simulink model "Logic_Final_Project_PRODUCT4_QUESTION37"  (R2025b)
settings: Solver=VariableStepAuto  StartTime=0.0  StopTime=100  RelTol=1e-3
libraries: simulink_extras x83
(part 1 of 2)
settings Model: Creator=60nur  LastModifiedBy=yusuf

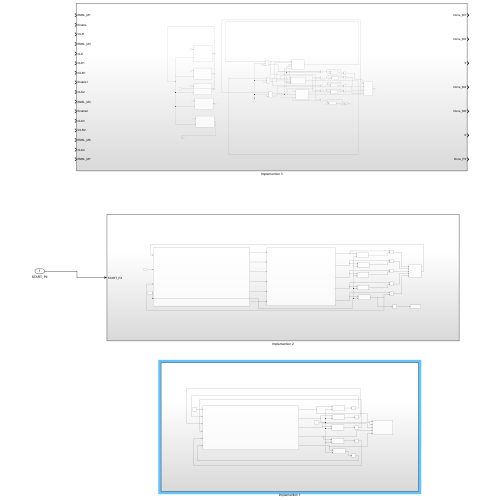
[thumbnail: Simulink's stored preview of the top-level diagram]
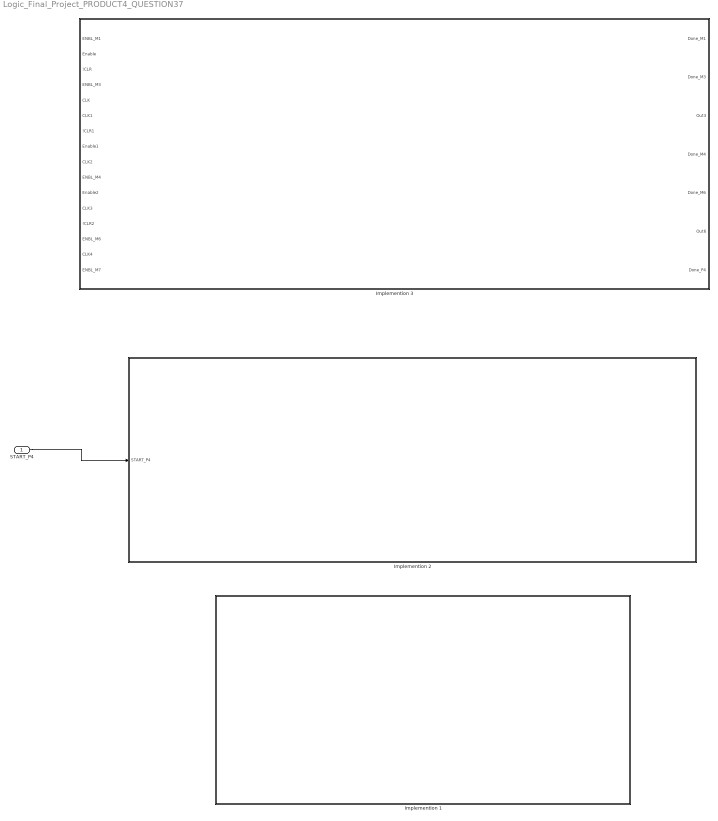
== system Logic_Final_Project_PRODUCT4_QUESTION37 ==
  START_P4 : Inport
  Implemention 1 : Subsystem
  Implemention 2 : Subsystem
  Implemention 3 : Subsystem
  wires:
  START_P4/1 -> Implemention 2/1(START_P4)

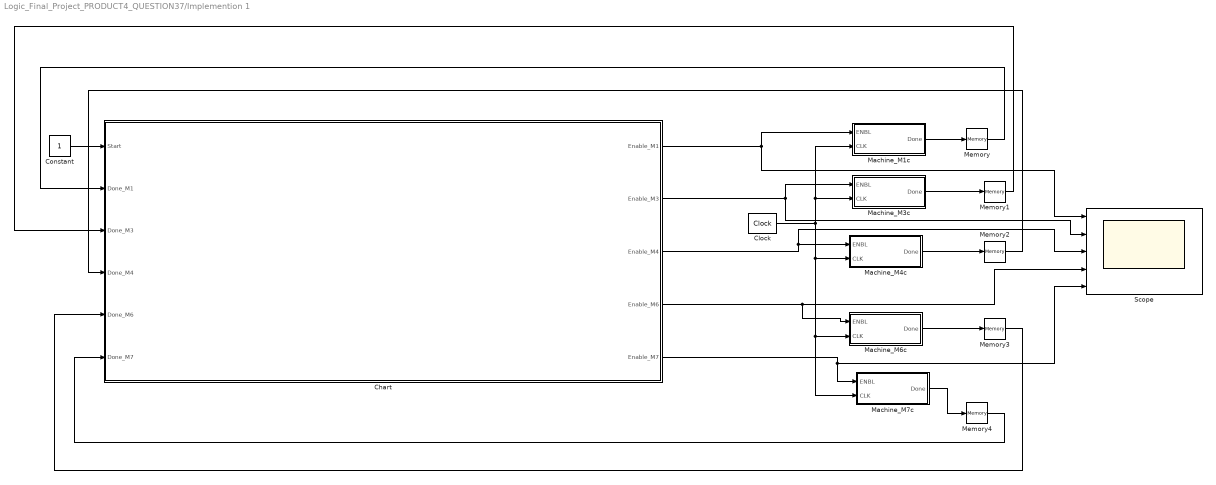
== system Logic_Final_Project_PRODUCT4_QUESTION37/Implemention 1 ==
  Chart : Stateflow chart  TreatAsAtomicUnit=on
  Clock : simulink_extras/Flip Flops/Clock  period=1
  Constant : Constant
  Machine_M1c : Subsystem
  Machine_M3c : Subsystem
  Machine_M4c : Subsystem
  Machine_M6c : Subsystem
  Machine_M7c : Subsystem
  Memory{,1..4} (5 alike) : Memory
  Scope : Scope  NumInputPorts=5
      settings: ActiveDisplayYMinimum=-0.1598262181001921  ActiveDisplayYMaximum=0.46246359997809955
  wires:
  Chart/5(Enable_M7) -> Machine_M7c/1(ENBL), Scope/5
  Chart/3(Enable_M4) -> Machine_M4c/1(ENBL), Scope/3
  Chart/4(Enable_M6) -> Machine_M6c/1(ENBL), Scope/4
  Memory3/1 -> Chart/5(Done_M6)
  Machine_M4c/1(Done) -> Memory2/1
  Machine_M3c/1(Done) -> Memory1/1
  Memory1/1 -> Chart/3(Done_M3)
  Memory4/1 -> Chart/6(Done_M7)
  Chart/2(Enable_M3) -> Machine_M3c/1(ENBL), Scope/2
  Chart/1(Enable_M1) -> Machine_M1c/1(ENBL), Scope/1
  Machine_M1c/1(Done) -> Memory/1
  Memory2/1 -> Chart/4(Done_M4)
  Clock/1 -> Machine_M1c/2(CLK), Machine_M3c/2(CLK), Machine_M7c/2(CLK), Machine_M6c/2(CLK), Machine_M4c/2(CLK)
  Constant/1 -> Chart/1(Start)
  Memory/1 -> Chart/2(Done_M1)
  Machine_M7c/1(Done) -> Memory4/1
  Machine_M6c/1(Done) -> Memory3/1

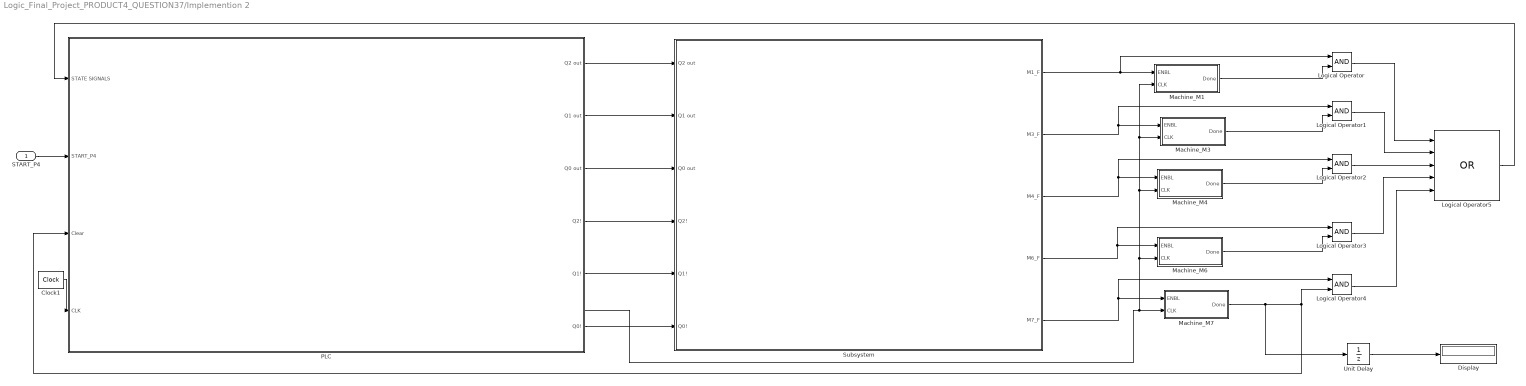
== system Logic_Final_Project_PRODUCT4_QUESTION37/Implemention 2 ==
  START_P4 : Inport
  Clock1 : simulink_extras/Flip Flops/Clock  period=1
  Display : Display
  Logical Operator{,1..4} (5 alike) : Logic  AllPortsSameDT=off  OutDataTypeStr=boolean
  Logical Operator5 : Logic  Operator=OR  Inputs=5  AllPortsSameDT=off  OutDataTypeStr=boolean
  Machine_M1 : Subsystem
  Machine_M3 : Subsystem
  Machine_M4 : Subsystem
  Machine_M6 : Subsystem
  Machine_M7 : Subsystem
  PLC : Subsystem
  Subsystem : Subsystem
  Unit Delay : UnitDelay  SampleTime=-1  HasFrameUpgradeWarning=on
  wires:
  Clock1/1 -> PLC/4(CLK), Machine_M6/2(CLK), Machine_M1/2(CLK), Machine_M3/2(CLK), Machine_M4/2(CLK), Machine_M7/2(CLK)
  PLC/1(Q2 out) -> Subsystem/1(Q2 out)
  Machine_M6/1(Done) -> Logical Operator3/2
  Subsystem/1(M1_F) -> Logical Operator/1, Machine_M1/1(ENBL)
  Subsystem/2(M3_F) -> Logical Operator1/1, Machine_M3/1(ENBL)
  Logical Operator/1 -> Logical Operator5/1
  Machine_M7/1(Done) -> Unit Delay/1, PLC/3(Clear), Logical Operator4/2
  Logical Operator4/1 -> Logical Operator5/5
  Logical Operator2/1 -> Logical Operator5/3
  Logical Operator3/1 -> Logical Operator5/4
  PLC/2(Q1 out) -> Subsystem/2(Q1 out)
  PLC/6(Q0!) -> Subsystem/6(Q0!)
  Unit Delay/1 -> Display/1
  Machine_M4/1(Done) -> Logical Operator2/2
  Subsystem/5(M7_F) -> Logical Operator4/1, Machine_M7/1(ENBL)
  PLC/5(Q1!) -> Subsystem/5(Q1!)
  Subsystem/3(M4_F) -> Logical Operator2/1, Machine_M4/1(ENBL)
  Subsystem/4(M6_F) -> Logical Operator3/1, Machine_M6/1(ENBL)
  PLC/4(Q2!) -> Subsystem/4(Q2!)
  PLC/3(Q0 out) -> Subsystem/3(Q0 out)
  START_P4/1 -> PLC/2(START_P4)
  Machine_M3/1(Done) -> Logical Operator1/2
  Logical Operator1/1 -> Logical Operator5/2
  Machine_M1/1(Done) -> Logical Operator/2
  Logical Operator5/1 -> PLC/1("STATE SIGNALS ")

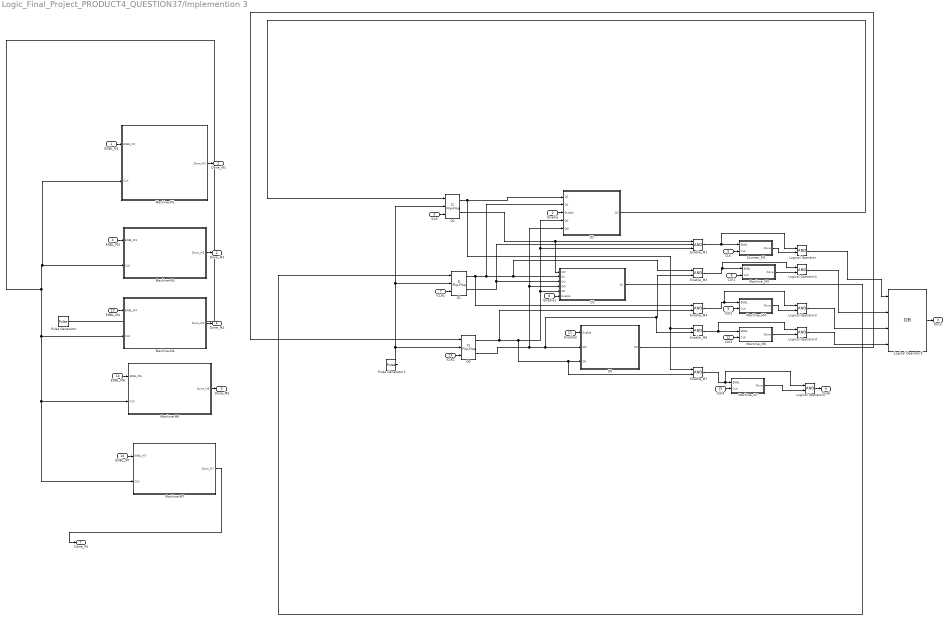
== system Logic_Final_Project_PRODUCT4_QUESTION37/Implemention 3 ==
  ENBL_M1 : Inport
  Enable : Inport  Port=2
  !CLR : Inport  Port=3
  ENBL_M3 : Inport  Port=4
  CLK : Inport  Port=5
  CLK1 : Inport  Port=6
  !CLR1 : Inport  Port=7
  Enable1 : Inport  Port=8
  CLK2 : Inport  Port=9
  ENBL_M4 : Inport  Port=10
  Enable2 : Inport  Port=11
  CLK3 : Inport  Port=12
  !CLR2 : Inport  Port=13
  ENBL_M6 : Inport  Port=14
  CLK4 : Inport  Port=15
  ENBL_M7 : Inport  Port=16
  Counter_M1 : Subsystem
  D0 : Subsystem
  D1 : Subsystem
  "D2 " : Subsystem
  Enable_M1 : Logic  Inputs=3  AllPortsSameDT=off  OutDataTypeStr=boolean
  Enable_M{3..4,6..7} (4 alike) : Logic  AllPortsSameDT=off  OutDataTypeStr=boolean
  Logical Operator{,1..4} (5 alike) : Logic  AllPortsSameDT=off  OutDataTypeStr=boolean
  Logical Operator5 : Logic  Operator=OR  Inputs=4  AllPortsSameDT=off  OutDataTypeStr=boolean
  Machine-M1 : Subsystem
  Machine-M3 : Subsystem
  Machine-M4 : Subsystem
  Machine-M6 : Subsystem
  Machine-M7 : Subsystem
  Machine_M3 : Subsystem
  Machine_M4 : Subsystem
  Machine_M6 : Subsystem
  Machine_M7 : Subsystem
  Pulse Generator : DiscretePulseGenerator  Period=10  PulseWidth=5  SampleTime=-1
  Pulse Generator1 : DiscretePulseGenerator  Period=10  PulseWidth=5  SampleTime=-1
  Q0 : simulink_extras/Flip Flops/D Flip-Flop
  Q1 : simulink_extras/Flip Flops/D Flip-Flop
  Q2 : simulink_extras/Flip Flops/D Flip-Flop
  Done_M1 : Outport
  Done_M3 : Outport  Port=2
  Out3 : Outport  Port=3
  Done_M4 : Outport  Port=4
  Done_M6 : Outport  Port=5
  Out6 : Outport  Port=6
  Done_P4 : Outport  Port=7
  wires:
  Machine_M7/1(Done) -> Logical Operator4/2
  Pulse Generator/1 -> Machine-M1/2(CLK), Machine-M3/2(CLK), Machine-M4/2(CLK), Machine-M7/2(CLK), Machine-M6/2(CLK)
  Q0/1 -> Enable_M4/2, D1/5(Q0), Enable_M1/3, "D2 "/4(Q0), Enable_M7/2, D0/3(Q0)
  Q2/1 -> Enable_M6/1, Enable_M7/1, "D2 "/1(Q2)
  Q1/1 -> Enable_M4/1, Enable_M3/1, D1/2(Q1), "D2 "/2(Q1)
  Enable_M7/1 -> Logical Operator4/1, Machine_M7/1(ENBL)
  Logical Operator2/1 -> Logical Operator5/3
  Machine_M6/1(Done) -> Logical Operator3/2
  Q1/2 -> Enable_M1/2, D1/3(Q1!)
  CLK4/1 -> Machine_M7/2(CLK)
  Enable_M3/1 -> Logical Operator1/1, Machine_M3/1(ENBL)
  Q2/2 -> Enable_M1/1, D1/1(Q2!)
  Logical Operator/1 -> Logical Operator5/1
  Machine-M7/1(Done_M7) -> Done_P4/1
  Enable_M4/1 -> Logical Operator2/1, Machine_M4/1(ENBL)
  Machine_M3/1(Done) -> Logical Operator1/2
  Pulse Generator1/1 -> Q0/2, Q1/2, Q2/2
  Enable/1 -> "D2 "/3(Enable)
  "D2 "/1(D2) -> Q2/1
  Machine-M3/1(Done_M3) -> Done_M3/1
  ENBL_M3/1 -> Machine-M3/1(ENBL_M3)
  D1/1(D1) -> Q1/1
  D0/1(D0) -> Q0/1
  Enable_M6/1 -> Logical Operator3/1, Machine_M6/1(ENBL)
  ENBL_M4/1 -> Machine-M4/1(ENBL_M4)
  Logical Operator5/1 -> Out3/1
  Counter_M1/1(Done) -> Logical Operator/2
  Enable_M1/1 -> Logical Operator/1, Counter_M1/1(ENBL)
  Logical Operator1/1 -> Logical Operator5/2
  ENBL_M1/1 -> Machine-M1/1(ENBL_M1)
  Machine_M4/1(Done) -> Logical Operator2/2
  Logical Operator3/1 -> Logical Operator5/4
  Q0/2 -> D0/2(Q0!), Enable_M6/2, Enable_M3/2, "D2 "/5(Q0!), D1/4(Q0!)
  CLK/1 -> Counter_M1/2(CLK)
  ENBL_M6/1 -> Machine-M6/1(ENBL_M6)
  CLK1/1 -> Machine_M3/2(CLK)
  Enable2/1 -> D0/1(Enable)
  !CLR1/1 -> Q1/3
  Machine-M6/1(Done_M6) -> Done_M6/1
  !CLR/1 -> Q2/3
  !CLR2/1 -> Q0/3
  Machine-M1/1(Done_M1) -> Done_M1/1
  Enable1/1 -> D1/6(Enable)
  CLK2/1 -> Machine_M4/2(CLK)
  Machine-M4/1(Done_M4) -> Done_M4/1
  CLK3/1 -> Machine_M6/2(CLK)
  ENBL_M7/1 -> Machine-M7/1(ENBL_M7)
  Logical Operator4/1 -> Out6/1

== system Logic_Final_Project_PRODUCT4_QUESTION37/Implemention 1/Machine_M1c ==
  ENBL : Inport
  CLK : Inport  Port=2
  D Flip-Flop 0 : simulink_extras/Flip Flops/D Flip-Flop
  D Flip-Flop1 : simulink_extras/Flip Flops/D Flip-Flop
  D Flip-Flop2 : simulink_extras/Flip Flops/D Flip-Flop
  Logical Operator : Logic  Operator=XOR  AllPortsSameDT=off  OutDataTypeStr=boolean
  Logical Operator1 : Logic  AllPortsSameDT=off  OutDataTypeStr=boolean
  Logical Operator2 : Logic  AllPortsSameDT=off  OutDataTypeStr=boolean
  Logical Operator3 : Logic  Operator=XOR  AllPortsSameDT=off  OutDataTypeStr=boolean
  Done : Outport
  wires:
  D Flip-Flop 0/2 -> D Flip-Flop 0/1
  D Flip-Flop 0/1 -> Logical Operator1/1, Logical Operator/1, Logical Operator2/1
  D Flip-Flop1/1 -> Logical Operator1/2, Logical Operator/2
  Logical Operator/1 -> D Flip-Flop1/1
  Logical Operator1/1 -> Logical Operator3/1
  D Flip-Flop2/1 -> Logical Operator2/2, Logical Operator3/2
  Logical Operator3/1 -> D Flip-Flop2/1
  ENBL/1 -> D Flip-Flop 0/3, D Flip-Flop2/3, D Flip-Flop1/3
  CLK/1 -> D Flip-Flop 0/2, D Flip-Flop1/2, D Flip-Flop2/2
  Logical Operator2/1 -> Done/1

== system Logic_Final_Project_PRODUCT4_QUESTION37/Implemention 1/Machine_M3c ==
  ENBL : Inport
  CLK : Inport  Port=2
  D Flip-Flop 0 : simulink_extras/Flip Flops/D Flip-Flop
  D Flip-Flop1 : simulink_extras/Flip Flops/D Flip-Flop
  D Flip-Flop2 : simulink_extras/Flip Flops/D Flip-Flop
  Logical Operator : Logic  Operator=XOR  AllPortsSameDT=off  OutDataTypeStr=boolean
  Logical Operator1 : Logic  AllPortsSameDT=off  OutDataTypeStr=boolean
  Logical Operator3 : Logic  Operator=XOR  AllPortsSameDT=off  OutDataTypeStr=boolean
  Done : Outport
  wires:
  CLK/1 -> D Flip-Flop2/2, D Flip-Flop1/2, D Flip-Flop 0/2
  ENBL/1 -> D Flip-Flop1/3, D Flip-Flop2/3, D Flip-Flop 0/3
  Logical Operator3/1 -> D Flip-Flop2/1
  D Flip-Flop2/1 -> Done/1, Logical Operator3/2
  Logical Operator1/1 -> Logical Operator3/1
  Logical Operator/1 -> D Flip-Flop1/1
  D Flip-Flop1/1 -> Logical Operator/2, Logical Operator1/2
  D Flip-Flop 0/1 -> Logical Operator/1, Logical Operator1/1
  D Flip-Flop 0/2 -> D Flip-Flop 0/1

== system Logic_Final_Project_PRODUCT4_QUESTION37/Implemention 1/Machine_M4c ==
  ENBL : Inport
  CLK : Inport  Port=2
  D Flip-Flop 0 : simulink_extras/Flip Flops/D Flip-Flop
  D Flip-Flop1 : simulink_extras/Flip Flops/D Flip-Flop
  D Flip-Flop2 : simulink_extras/Flip Flops/D Flip-Flop
  Logical Operator : Logic  Operator=XOR  AllPortsSameDT=off  OutDataTypeStr=boolean
  Logical Operator1 : Logic  AllPortsSameDT=off  OutDataTypeStr=boolean
  Logical Operator2 : Logic  AllPortsSameDT=off  OutDataTypeStr=boolean
  Logical Operator3 : Logic  Operator=XOR  AllPortsSameDT=off  OutDataTypeStr=boolean
  Done : Outport
  wires:
  Logical Operator2/1 -> Done/1
  CLK/1 -> D Flip-Flop2/2, D Flip-Flop1/2, D Flip-Flop 0/2
  ENBL/1 -> D Flip-Flop1/3, D Flip-Flop2/3, D Flip-Flop 0/3
  Logical Operator3/1 -> D Flip-Flop2/1
  D Flip-Flop2/1 -> Logical Operator3/2, Logical Operator2/2
  Logical Operator1/1 -> Logical Operator3/1
  Logical Operator/1 -> D Flip-Flop1/1
  D Flip-Flop1/1 -> Logical Operator/2, Logical Operator1/2
  D Flip-Flop 0/1 -> Logical Operator2/1, Logical Operator/1, Logical Operator1/1
  D Flip-Flop 0/2 -> D Flip-Flop 0/1

== system Logic_Final_Project_PRODUCT4_QUESTION37/Implemention 1/Machine_M6c ==
  ENBL : Inport
  CLK : Inport  Port=2
  D Flip-Flop 0 : simulink_extras/Flip Flops/D Flip-Flop
  D Flip-Flop1 : simulink_extras/Flip Flops/D Flip-Flop
  D Flip-Flop2 : simulink_extras/Flip Flops/D Flip-Flop
  Logical Operator : Logic  Operator=XOR  AllPortsSameDT=off  OutDataTypeStr=boolean
  Logical Operator1 : Logic  AllPortsSameDT=off  OutDataTypeStr=boolean
  Logical Operator2 : Logic  AllPortsSameDT=off  OutDataTypeStr=boolean
  Logical Operator3 : Logic  Operator=XOR  AllPortsSameDT=off  OutDataTypeStr=boolean
  Done : Outport
  wires:
  Logical Operator2/1 -> Done/1
  CLK/1 -> D Flip-Flop2/2, D Flip-Flop1/2, D Flip-Flop 0/2
  ENBL/1 -> D Flip-Flop1/3, D Flip-Flop2/3, D Flip-Flop 0/3
  Logical Operator3/1 -> D Flip-Flop2/1
  D Flip-Flop2/1 -> Logical Operator3/2, Logical Operator2/2
  Logical Operator1/1 -> Logical Operator3/1
  Logical Operator/1 -> D Flip-Flop1/1
  D Flip-Flop1/1 -> Logical Operator/2, Logical Operator1/2, Logical Operator2/1
  D Flip-Flop 0/1 -> Logical Operator/1, Logical Operator1/1
  D Flip-Flop 0/2 -> D Flip-Flop 0/1

== system Logic_Final_Project_PRODUCT4_QUESTION37/Implemention 1/Machine_M7c ==
  ENBL : Inport
  CLK : Inport  Port=2
  D Flip-Flop 0 : simulink_extras/Flip Flops/D Flip-Flop
  D Flip-Flop1 : simulink_extras/Flip Flops/D Flip-Flop
  D Flip-Flop2 : simulink_extras/Flip Flops/D Flip-Flop
  Logical Operator : Logic  Operator=XOR  AllPortsSameDT=off  OutDataTypeStr=boolean
  Logical Operator1 : Logic  AllPortsSameDT=off  OutDataTypeStr=boolean
  Logical Operator3 : Logic  Operator=XOR  AllPortsSameDT=off  OutDataTypeStr=boolean
  Done : Outport
  wires:
  D Flip-Flop 0/2 -> D Flip-Flop 0/1
  D Flip-Flop 0/1 -> Logical Operator1/1, Logical Operator/1
  D Flip-Flop1/1 -> Done/1, Logical Operator1/2, Logical Operator/2
  Logical Operator/1 -> D Flip-Flop1/1
  Logical Operator1/1 -> Logical Operator3/1
  D Flip-Flop2/1 -> Logical Operator3/2
  Logical Operator3/1 -> D Flip-Flop2/1
  ENBL/1 -> D Flip-Flop 0/3, D Flip-Flop2/3, D Flip-Flop1/3
  CLK/1 -> D Flip-Flop 0/2, D Flip-Flop1/2, D Flip-Flop2/2

== system Logic_Final_Project_PRODUCT4_QUESTION37/Implemention 2/Machine_M1 ==
  ENBL : Inport
  CLK : Inport  Port=2
  D Flip-Flop 0 : simulink_extras/Flip Flops/D Flip-Flop
  D Flip-Flop1 : simulink_extras/Flip Flops/D Flip-Flop
  D Flip-Flop2 : simulink_extras/Flip Flops/D Flip-Flop
  Logical Operator : Logic  Operator=XOR  AllPortsSameDT=off  OutDataTypeStr=boolean
  Logical Operator1 : Logic  AllPortsSameDT=off  OutDataTypeStr=boolean
  Logical Operator2 : Logic  AllPortsSameDT=off  OutDataTypeStr=boolean
  Logical Operator3 : Logic  Operator=XOR  AllPortsSameDT=off  OutDataTypeStr=boolean
  Done : Outport
  wires:
  D Flip-Flop 0/2 -> D Flip-Flop 0/1
  D Flip-Flop 0/1 -> Logical Operator1/1, Logical Operator/1, Logical Operator2/1
  D Flip-Flop1/1 -> Logical Operator1/2, Logical Operator/2
  Logical Operator/1 -> D Flip-Flop1/1
  Logical Operator1/1 -> Logical Operator3/1
  D Flip-Flop2/1 -> Logical Operator2/2, Logical Operator3/2
  Logical Operator3/1 -> D Flip-Flop2/1
  ENBL/1 -> D Flip-Flop 0/3, D Flip-Flop2/3, D Flip-Flop1/3
  CLK/1 -> D Flip-Flop 0/2, D Flip-Flop1/2, D Flip-Flop2/2
  Logical Operator2/1 -> Done/1

== system Logic_Final_Project_PRODUCT4_QUESTION37/Implemention 2/Machine_M3 ==
  ENBL : Inport
  CLK : Inport  Port=2
  D Flip-Flop 0 : simulink_extras/Flip Flops/D Flip-Flop
  D Flip-Flop1 : simulink_extras/Flip Flops/D Flip-Flop
  D Flip-Flop2 : simulink_extras/Flip Flops/D Flip-Flop
  Logical Operator : Logic  Operator=XOR  AllPortsSameDT=off  OutDataTypeStr=boolean
  Logical Operator1 : Logic  AllPortsSameDT=off  OutDataTypeStr=boolean
  Logical Operator3 : Logic  Operator=XOR  AllPortsSameDT=off  OutDataTypeStr=boolean
  Done : Outport
  wires:
  CLK/1 -> D Flip-Flop2/2, D Flip-Flop1/2, D Flip-Flop 0/2
  ENBL/1 -> D Flip-Flop1/3, D Flip-Flop2/3, D Flip-Flop 0/3
  Logical Operator3/1 -> D Flip-Flop2/1
  D Flip-Flop2/1 -> Done/1, Logical Operator3/2
  Logical Operator1/1 -> Logical Operator3/1
  Logical Operator/1 -> D Flip-Flop1/1
  D Flip-Flop1/1 -> Logical Operator/2, Logical Operator1/2
  D Flip-Flop 0/1 -> Logical Operator/1, Logical Operator1/1
  D Flip-Flop 0/2 -> D Flip-Flop 0/1

== system Logic_Final_Project_PRODUCT4_QUESTION37/Implemention 2/Machine_M4 ==
  ENBL : Inport
  CLK : Inport  Port=2
  D Flip-Flop 0 : simulink_extras/Flip Flops/D Flip-Flop
  D Flip-Flop1 : simulink_extras/Flip Flops/D Flip-Flop
  D Flip-Flop2 : simulink_extras/Flip Flops/D Flip-Flop
  Logical Operator : Logic  Operator=XOR  AllPortsSameDT=off  OutDataTypeStr=boolean
  Logical Operator1 : Logic  AllPortsSameDT=off  OutDataTypeStr=boolean
  Logical Operator2 : Logic  AllPortsSameDT=off  OutDataTypeStr=boolean
  Logical Operator3 : Logic  Operator=XOR  AllPortsSameDT=off  OutDataTypeStr=boolean
  Done : Outport
  wires:
  Logical Operator2/1 -> Done/1
  CLK/1 -> D Flip-Flop2/2, D Flip-Flop1/2, D Flip-Flop 0/2
  ENBL/1 -> D Flip-Flop1/3, D Flip-Flop2/3, D Flip-Flop 0/3
  Logical Operator3/1 -> D Flip-Flop2/1
  D Flip-Flop2/1 -> Logical Operator3/2, Logical Operator2/2
  Logical Operator1/1 -> Logical Operator3/1
  Logical Operator/1 -> D Flip-Flop1/1
  D Flip-Flop1/1 -> Logical Operator/2, Logical Operator1/2
  D Flip-Flop 0/1 -> Logical Operator2/1, Logical Operator/1, Logical Operator1/1
  D Flip-Flop 0/2 -> D Flip-Flop 0/1

== system Logic_Final_Project_PRODUCT4_QUESTION37/Implemention 2/Machine_M6 ==
  ENBL : Inport
  CLK : Inport  Port=2
  D Flip-Flop 0 : simulink_extras/Flip Flops/D Flip-Flop
  D Flip-Flop1 : simulink_extras/Flip Flops/D Flip-Flop
  D Flip-Flop2 : simulink_extras/Flip Flops/D Flip-Flop
  Logical Operator : Logic  Operator=XOR  AllPortsSameDT=off  OutDataTypeStr=boolean
  Logical Operator1 : Logic  AllPortsSameDT=off  OutDataTypeStr=boolean
  Logical Operator2 : Logic  AllPortsSameDT=off  OutDataTypeStr=boolean
  Logical Operator3 : Logic  Operator=XOR  AllPortsSameDT=off  OutDataTypeStr=boolean
  Done : Outport
  wires:
  Logical Operator2/1 -> Done/1
  CLK/1 -> D Flip-Flop2/2, D Flip-Flop1/2, D Flip-Flop 0/2
  ENBL/1 -> D Flip-Flop1/3, D Flip-Flop2/3, D Flip-Flop 0/3
  Logical Operator3/1 -> D Flip-Flop2/1
  D Flip-Flop2/1 -> Logical Operator3/2, Logical Operator2/2
  Logical Operator1/1 -> Logical Operator3/1
  Logical Operator/1 -> D Flip-Flop1/1
  D Flip-Flop1/1 -> Logical Operator/2, Logical Operator1/2, Logical Operator2/1
  D Flip-Flop 0/1 -> Logical Operator/1, Logical Operator1/1
  D Flip-Flop 0/2 -> D Flip-Flop 0/1

== system Logic_Final_Project_PRODUCT4_QUESTION37/Implemention 2/Machine_M7 ==
  ENBL : Inport
  CLK : Inport  Port=2
  D Flip-Flop 0 : simulink_extras/Flip Flops/D Flip-Flop
  D Flip-Flop1 : simulink_extras/Flip Flops/D Flip-Flop
  D Flip-Flop2 : simulink_extras/Flip Flops/D Flip-Flop
  Logical Operator : Logic  Operator=XOR  AllPortsSameDT=off  OutDataTypeStr=boolean
  Logical Operator1 : Logic  AllPortsSameDT=off  OutDataTypeStr=boolean
  Logical Operator3 : Logic  Operator=XOR  AllPortsSameDT=off  OutDataTypeStr=boolean
  Unit Delay : UnitDelay  SampleTime=-1  HasFrameUpgradeWarning=on
  Done : Outport
  wires:
  D Flip-Flop 0/2 -> D Flip-Flop 0/1
  D Flip-Flop 0/1 -> Logical Operator1/1, Logical Operator/1
  Logical Operator1/1 -> Logical Operator3/1
  D Flip-Flop2/1 -> Logical Operator3/2
  Logical Operator3/1 -> D Flip-Flop2/1
  ENBL/1 -> D Flip-Flop 0/3, D Flip-Flop2/3, D Flip-Flop1/3
  CLK/1 -> D Flip-Flop 0/2, D Flip-Flop1/2, D Flip-Flop2/2
  Logical Operator/1 -> D Flip-Flop1/1
  D Flip-Flop1/1 -> Unit Delay/1
  Unit Delay/1 -> Done/1, Logical Operator/2, Logical Operator1/2

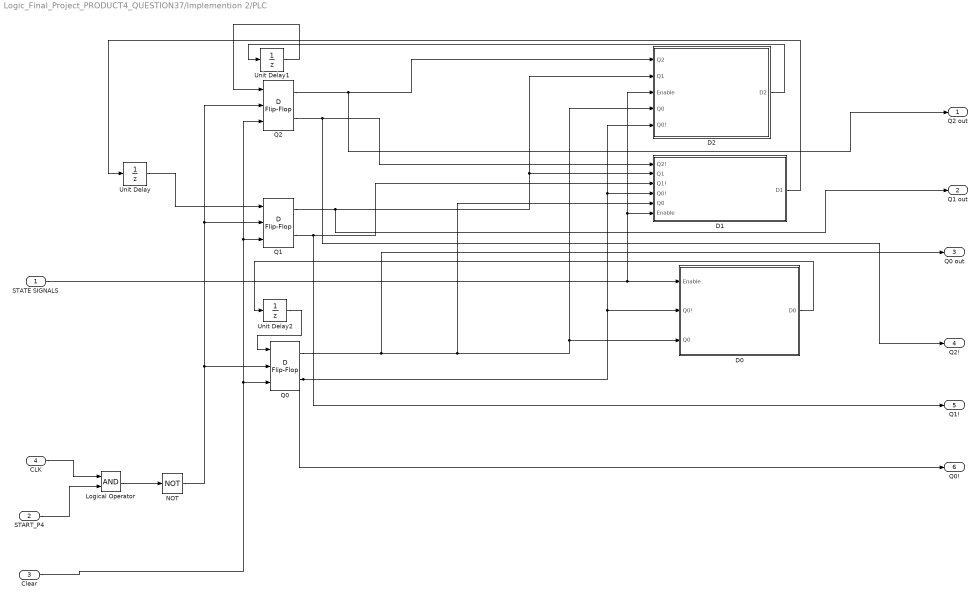
== system Logic_Final_Project_PRODUCT4_QUESTION37/Implemention 2/PLC ==
  "STATE SIGNALS " : Inport
  START_P4 : Inport  Port=2
  Clear : Inport  Port=3
  CLK : Inport  Port=4
  D0 : Subsystem
  D1 : Subsystem
  "D2 " : Subsystem
  Logical Operator : Logic  AllPortsSameDT=off  OutDataTypeStr=boolean
  NOT : Logic  Operator=NOT  IconShape=distinctive  AllPortsSameDT=off  OutDataTypeStr=boolean
  Q0 : simulink_extras/Flip Flops/D Flip-Flop
  Q1 : simulink_extras/Flip Flops/D Flip-Flop
  Q2 : simulink_extras/Flip Flops/D Flip-Flop
  Unit Delay : UnitDelay  SampleTime=-1  HasFrameUpgradeWarning=on
  Unit Delay1 : UnitDelay  SampleTime=-1  HasFrameUpgradeWarning=on
  Unit Delay2 : UnitDelay  SampleTime=-1  HasFrameUpgradeWarning=on
  Q2 out : Outport
  Q1 out : Outport  Port=2
  Q0 out : Outport  Port=3
  Q2! : Outport  Port=4
  Q1! : Outport  Port=5
  Q0! : Outport  Port=6
  wires:
  Q2/1 -> Q2 out/1, "D2 "/1(Q2)
  Q1/1 -> Q1 out/1, "D2 "/2(Q1), D1/2(Q1)
  Q0/1 -> Q0 out/1, D1/5(Q0), "D2 "/4(Q0), D0/3(Q0)
  Q0/2 -> Q0!/1, "D2 "/5(Q0!), D1/4(Q0!), D0/2(Q0!)
  Q2/2 -> Q2!/1, D1/1(Q2!)
  Q1/2 -> Q1!/1, D1/3(Q1!)
  Logical Operator/1 -> NOT/1
  CLK/1 -> Logical Operator/1
  NOT/1 -> Q0/2, Q2/2, Q1/2
  "STATE SIGNALS "/1 -> "D2 "/3(Enable), D1/6(Enable), D0/1(Enable)
  Clear/1 -> Q2/3, Q1/3, Q0/3
  Unit Delay2/1 -> Q0/1
  D0/1(D0) -> Unit Delay2/1
  Unit Delay1/1 -> Q2/1
  "D2 "/1(D2) -> Unit Delay1/1
  Unit Delay/1 -> Q1/1
  D1/1(D1) -> Unit Delay/1
  START_P4/1 -> Logical Operator/2

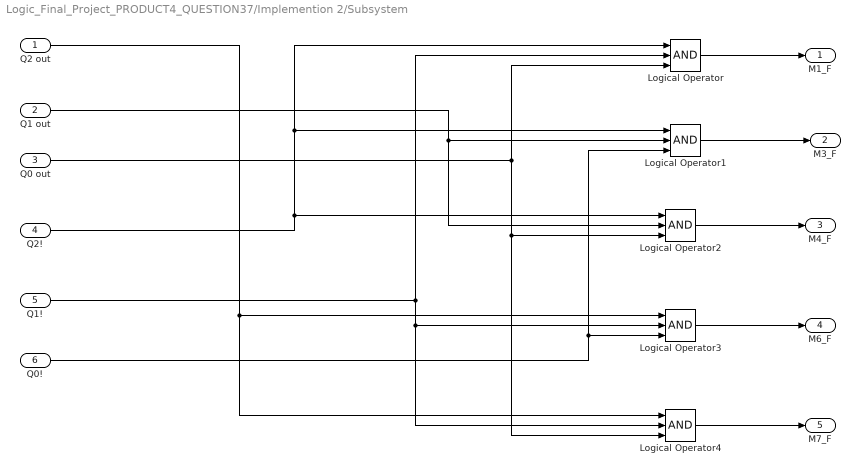
== system Logic_Final_Project_PRODUCT4_QUESTION37/Implemention 2/Subsystem ==
  Q2 out : Inport
  Q1 out : Inport  Port=2
  Q0 out : Inport  Port=3
  Q2! : Inport  Port=4
  Q1! : Inport  Port=5
  Q0! : Inport  Port=6
  Logical Operator{,1..4} (5 alike) : Logic  Inputs=3  AllPortsSameDT=off  OutDataTypeStr=boolean
  M1_F : Outport
  M3_F : Outport  Port=2
  M4_F : Outport  Port=3
  M6_F : Outport  Port=4
  M7_F : Outport  Port=5
  wires:
  Logical Operator2/1 -> M4_F/1
  Logical Operator4/1 -> M7_F/1
  Logical Operator3/1 -> M6_F/1
  Logical Operator1/1 -> M3_F/1
  Logical Operator/1 -> M1_F/1
  Q2!/1 -> Logical Operator2/1, Logical Operator1/1, Logical Operator/1
  Q1!/1 -> Logical Operator3/2, Logical Operator4/2, Logical Operator/2
  Q0 out/1 -> Logical Operator2/3, Logical Operator4/3, Logical Operator/3
  Q1 out/1 -> Logical Operator2/2, Logical Operator1/2
  Q0!/1 -> Logical Operator1/3, Logical Operator3/3
  Q2 out/1 -> Logical Operator4/1, Logical Operator3/1

== system Logic_Final_Project_PRODUCT4_QUESTION37/Implemention 3/Counter_M1 ==
  ENBL : Inport
  CLK : Inport  Port=2
  D Flip-Flop 0 : simulink_extras/Flip Flops/D Flip-Flop
  D Flip-Flop1 : simulink_extras/Flip Flops/D Flip-Flop
  D Flip-Flop2 : simulink_extras/Flip Flops/D Flip-Flop
  Logical Operator : Logic  Operator=XOR  AllPortsSameDT=off  OutDataTypeStr=boolean
  Logical Operator1 : Logic  AllPortsSameDT=off  OutDataTypeStr=boolean
  Logical Operator2 : Logic  AllPortsSameDT=off  OutDataTypeStr=boolean
  Logical Operator3 : Logic  Operator=XOR  AllPortsSameDT=off  OutDataTypeStr=boolean
  Done : Outport
  wires:
  D Flip-Flop 0/2 -> D Flip-Flop 0/1
  D Flip-Flop 0/1 -> Logical Operator1/1, Logical Operator/1, Logical Operator2/1
  D Flip-Flop1/1 -> Logical Operator1/2, Logical Operator/2
  Logical Operator/1 -> D Flip-Flop1/1
  Logical Operator1/1 -> Logical Operator3/1
  D Flip-Flop2/1 -> Logical Operator2/2, Logical Operator3/2
  Logical Operator3/1 -> D Flip-Flop2/1
  ENBL/1 -> D Flip-Flop 0/3, D Flip-Flop2/3, D Flip-Flop1/3
  CLK/1 -> D Flip-Flop 0/2, D Flip-Flop1/2, D Flip-Flop2/2
  Logical Operator2/1 -> Done/1

== system Logic_Final_Project_PRODUCT4_QUESTION37/Implemention 3/D0 ==
  Enable : Inport
  Q0! : Inport  Port=2
  Q0 : Inport  Port=3
  Logical Operator : Logic  AllPortsSameDT=off  OutDataTypeStr=boolean
  Logical Operator1 : Logic  Operator=NOT  AllPortsSameDT=off  OutDataTypeStr=boolean
  Logical Operator2 : Logic  Operator=OR  AllPortsSameDT=off  OutDataTypeStr=boolean
  Logical Operator3 : Logic  AllPortsSameDT=off  OutDataTypeStr=boolean
  D0 : Outport
  wires:
  Logical Operator1/1 -> Logical Operator/2
  Logical Operator/1 -> Logical Operator2/2
  Logical Operator2/1 -> D0/1
  Logical Operator3/1 -> Logical Operator2/1
  Enable/1 -> Logical Operator1/1, Logical Operator3/1
  Q0!/1 -> Logical Operator3/2
  Q0/1 -> Logical Operator/1

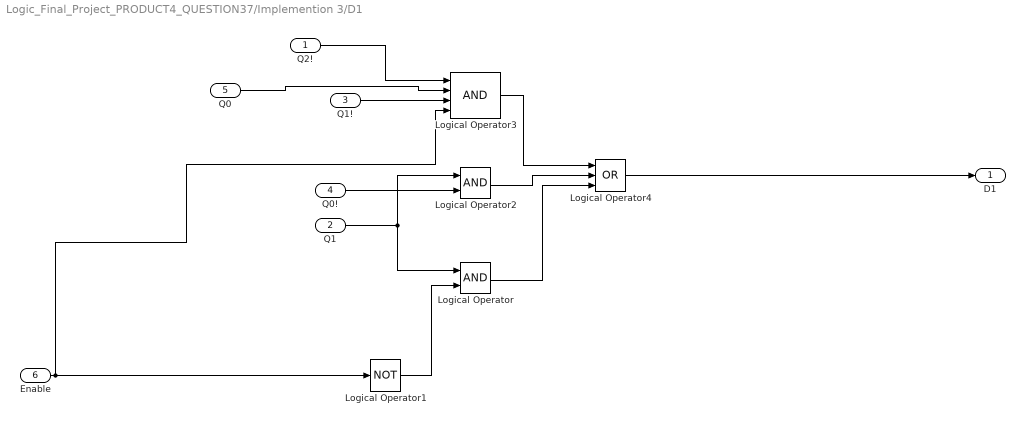
== system Logic_Final_Project_PRODUCT4_QUESTION37/Implemention 3/D1 ==
  Q2! : Inport
  Q1 : Inport  Port=2
  Q1! : Inport  Port=3
  Q0! : Inport  Port=4
  Q0 : Inport  Port=5
  Enable : Inport  Port=6
  Logical Operator : Logic  AllPortsSameDT=off  OutDataTypeStr=boolean
  Logical Operator1 : Logic  Operator=NOT  AllPortsSameDT=off  OutDataTypeStr=boolean
  Logical Operator2 : Logic  AllPortsSameDT=off  OutDataTypeStr=boolean
  Logical Operator3 : Logic  Inputs=4  AllPortsSameDT=off  OutDataTypeStr=boolean
  Logical Operator4 : Logic  Operator=OR  Inputs=3  AllPortsSameDT=off  OutDataTypeStr=boolean
  D1 : Outport
  wires:
  Q0/1 -> Logical Operator3/2
  Logical Operator1/1 -> Logical Operator/2
  Q1!/1 -> Logical Operator3/3
  Q1/1 -> Logical Operator2/1, Logical Operator/1
  Enable/1 -> Logical Operator3/4, Logical Operator1/1
  Q2!/1 -> Logical Operator3/1
  Q0!/1 -> Logical Operator2/2
  Logical Operator3/1 -> Logical Operator4/1
  Logical Operator2/1 -> Logical Operator4/2
  Logical Operator/1 -> Logical Operator4/3
  Logical Operator4/1 -> D1/1

== system Logic_Final_Project_PRODUCT4_QUESTION37/Implemention 3/D2  ==
  Q2 : Inport
  Q1 : Inport  Port=2
  Enable : Inport  Port=3
  Q0 : Inport  Port=4
  Q0! : Inport  Port=5
  Logical Operator : Logic  Operator=NOT  AllPortsSameDT=off  OutDataTypeStr=boolean
  Logical Operator1 : Logic  AllPortsSameDT=off  OutDataTypeStr=boolean
  Logical Operator2 : Logic  AllPortsSameDT=off  OutDataTypeStr=boolean
  Logical Operator3 : Logic  Inputs=3  AllPortsSameDT=off  OutDataTypeStr=boolean
  Logical Operator4 : Logic  Operator=OR  Inputs=3  AllPortsSameDT=off  OutDataTypeStr=boolean
  D2 : Outport
  wires:
  Q0/1 -> Logical Operator3/2
  Q2/1 -> Logical Operator2/1, Logical Operator1/1
  Q1/1 -> Logical Operator3/1
  Logical Operator3/1 -> Logical Operator4/3
  Logical Operator/1 -> Logical Operator1/2
  Logical Operator1/1 -> Logical Operator4/2
  Logical Operator2/1 -> Logical Operator4/1
  Enable/1 -> Logical Operator/1, Logical Operator3/3
  Q0!/1 -> Logical Operator2/2
  Logical Operator4/1 -> D2/1

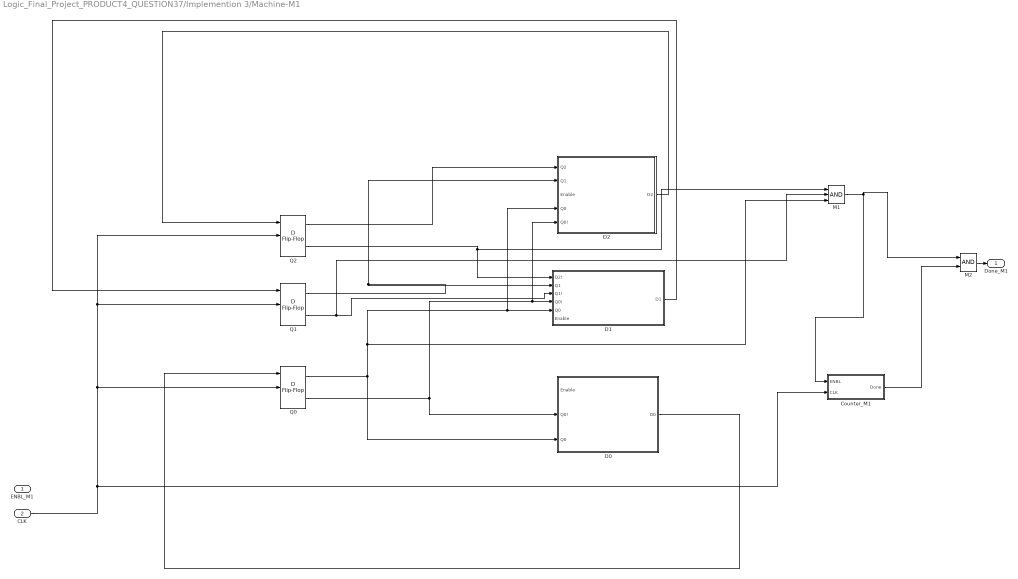
== system Logic_Final_Project_PRODUCT4_QUESTION37/Implemention 3/Machine-M1 ==
  ENBL_M1 : Inport
  CLK : Inport  Port=2
  Counter_M1 : Subsystem
  D0 : Subsystem
  D1 : Subsystem
  "D2 " : Subsystem
  M1 : Logic  Inputs=3  AllPortsSameDT=off  OutDataTypeStr=boolean
  M2 : Logic  AllPortsSameDT=off  OutDataTypeStr=boolean
  Q0 : simulink_extras/Flip Flops/D Flip-Flop
  Q1 : simulink_extras/Flip Flops/D Flip-Flop
  Q2 : simulink_extras/Flip Flops/D Flip-Flop
  Done_M1 : Outport
  wires:
  D0/1(D0) -> Q0/1
  Q2/2 -> D1/1(Q2!), M1/1
  Q1/1 -> D1/2(Q1), "D2 "/2(Q1)
  Q0/2 -> "D2 "/5(Q0!), D1/4(Q0!), D0/2(Q0!)
  Counter_M1/1(Done) -> M2/2
  D1/1(D1) -> Q1/1
  Q1/2 -> D1/3(Q1!), M1/2
  Q0/1 -> "D2 "/4(Q0), D1/5(Q0), M1/3, D0/3(Q0)
  M1/1 -> M2/1, Counter_M1/1(ENBL)
  Q2/1 -> "D2 "/1(Q2)
  "D2 "/1(D2) -> Q2/1
  M2/1 -> Done_M1/1
  CLK/1 -> Counter_M1/2(CLK), Q0/2, Q1/2, Q2/2

== system Logic_Final_Project_PRODUCT4_QUESTION37/Implemention 3/Machine-M3 ==
  ENBL_M3 : Inport
  CLK : Inport  Port=2
  D0 : Subsystem
  D1 : Subsystem
  "D2 " : Subsystem
  Logical Operator : Logic  Inputs=3  AllPortsSameDT=off  OutDataTypeStr=boolean
  Machine_M3 : Subsystem
  Q0 : simulink_extras/Flip Flops/D Flip-Flop
  Q1 : simulink_extras/Flip Flops/D Flip-Flop
  Q2 : simulink_extras/Flip Flops/D Flip-Flop
  Done_M3 : Outport
  wires:
  Logical Operator/1 -> Done_M3/1
  D0/1(D0) -> Q0/1
  D1/1(D1) -> Q1/1
  Q1/2 -> D1/3(Q1!)
  Q2/2 -> D1/1(Q2!)
  "D2 "/1(D2) -> Q2/1
  Q0/2 -> Logical Operator/2, D0/2(Q0!), D1/4(Q0!), "D2 "/5(Q0!)
  Q0/1 -> D0/3(Q0), "D2 "/4(Q0), D1/5(Q0)
  Q1/1 -> Logical Operator/1, D1/2(Q1), "D2 "/2(Q1)
  Q2/1 -> "D2 "/1(Q2)
  CLK/1 -> Machine_M3/2(CLK), Q0/2, Q2/2, Q1/2
  ENBL_M3/1 -> Machine_M3/1(ENBL), D0/1(Enable), D1/6(Enable), Q0/3, Q1/3, "D2 "/3(Enable), Q2/3
  Machine_M3/1(Done) -> Logical Operator/3

== system Logic_Final_Project_PRODUCT4_QUESTION37/Implemention 3/Machine-M4 ==
  ENBL_M4 : Inport
  CLK : Inport  Port=2
  D0 : Subsystem
  D1 : Subsystem
  "D2 " : Subsystem
  Logical Operator : Logic  Inputs=3  AllPortsSameDT=off  OutDataTypeStr=boolean
  Machine_M4 : Subsystem
  Q0 : simulink_extras/Flip Flops/D Flip-Flop
  Q1 : simulink_extras/Flip Flops/D Flip-Flop
  Q2 : simulink_extras/Flip Flops/D Flip-Flop
  Done_M4 : Outport
  wires:
  ENBL_M4/1 -> Machine_M4/1(ENBL), Q2/3, "D2 "/3(Enable), Q1/3, Q0/3, D1/6(Enable), D0/1(Enable)
  CLK/1 -> Machine_M4/2(CLK), Q1/2, Q2/2, Q0/2
  Q2/1 -> "D2 "/1(Q2)
  Q1/1 -> "D2 "/2(Q1), Logical Operator/1, D1/2(Q1)
  Q0/1 -> D1/5(Q0), Logical Operator/2, "D2 "/4(Q0), D0/3(Q0)
  Q0/2 -> "D2 "/5(Q0!), D1/4(Q0!), D0/2(Q0!)
  "D2 "/1(D2) -> Q2/1
  Q2/2 -> D1/1(Q2!)
  Q1/2 -> D1/3(Q1!)
  D1/1(D1) -> Q1/1
  D0/1(D0) -> Q0/1
  Logical Operator/1 -> Done_M4/1
  Machine_M4/1(Done) -> Logical Operator/3

== system Logic_Final_Project_PRODUCT4_QUESTION37/Implemention 3/Machine-M6 ==
  ENBL_M6 : Inport
  CLK : Inport  Port=2
  D0 : Subsystem
  D1 : Subsystem
  "D2 " : Subsystem
  Logical Operator : Logic  Inputs=3  AllPortsSameDT=off  OutDataTypeStr=boolean
  Machine_M6 : Subsystem
  Q0 : simulink_extras/Flip Flops/D Flip-Flop
  Q1 : simulink_extras/Flip Flops/D Flip-Flop
  Q2 : simulink_extras/Flip Flops/D Flip-Flop
  Done_M6 : Outport
  wires:
  Logical Operator/1 -> Done_M6/1
  D0/1(D0) -> Q0/1
  D1/1(D1) -> Q1/1
  Q1/2 -> D1/3(Q1!)
  Q2/2 -> D1/1(Q2!)
  "D2 "/1(D2) -> Q2/1
  Q0/2 -> Logical Operator/2, D0/2(Q0!), D1/4(Q0!), "D2 "/5(Q0!)
  Q0/1 -> D0/3(Q0), "D2 "/4(Q0), D1/5(Q0)
  Q1/1 -> D1/2(Q1), "D2 "/2(Q1)
  Q2/1 -> Logical Operator/1, "D2 "/1(Q2)
  CLK/1 -> Machine_M6/2(CLK), Q0/2, Q2/2, Q1/2
  ENBL_M6/1 -> Machine_M6/1(ENBL), D0/1(Enable), D1/6(Enable), Q0/3, Q1/3, "D2 "/3(Enable), Q2/3
  Machine_M6/1(Done) -> Logical Operator/3

== system Logic_Final_Project_PRODUCT4_QUESTION37/Implemention 3/Machine-M7 ==
  ENBL_M7 : Inport
  CLK : Inport  Port=2
  D0 : Subsystem
  D1 : Subsystem
  "D2 " : Subsystem
  Logical Operator : Logic  Inputs=3  AllPortsSameDT=off  OutDataTypeStr=boolean
  Machine_M7 : Subsystem
  Q0 : simulink_extras/Flip Flops/D Flip-Flop
  Q1 : simulink_extras/Flip Flops/D Flip-Flop
  Q2 : simulink_extras/Flip Flops/D Flip-Flop
  Done_M7 : Outport
  wires:
  ENBL_M7/1 -> Machine_M7/1(ENBL), Q2/3, "D2 "/3(Enable), Q1/3, Q0/3, D1/6(Enable), D0/1(Enable)
  CLK/1 -> Machine_M7/2(CLK), Q1/2, Q2/2, Q0/2
  Q2/1 -> Logical Operator/1, "D2 "/1(Q2)
  Q1/1 -> "D2 "/2(Q1), D1/2(Q1)
  Q0/1 -> D1/5(Q0), Logical Operator/2, "D2 "/4(Q0), D0/3(Q0)
  Q0/2 -> "D2 "/5(Q0!), D1/4(Q0!), D0/2(Q0!)
  "D2 "/1(D2) -> Q2/1
  Q2/2 -> D1/1(Q2!)
  Q1/2 -> D1/3(Q1!)
  D1/1(D1) -> Q1/1
  D0/1(D0) -> Q0/1
  Logical Operator/1 -> Done_M7/1
  Machine_M7/1(Done) -> Logical Operator/3

== system Logic_Final_Project_PRODUCT4_QUESTION37/Implemention 3/Machine_M3 ==
  ENBL : Inport
  CLK : Inport  Port=2
  D Flip-Flop 0 : simulink_extras/Flip Flops/D Flip-Flop
  D Flip-Flop1 : simulink_extras/Flip Flops/D Flip-Flop
  D Flip-Flop2 : simulink_extras/Flip Flops/D Flip-Flop
  Logical Operator : Logic  Operator=XOR  AllPortsSameDT=off  OutDataTypeStr=boolean
  Logical Operator1 : Logic  AllPortsSameDT=off  OutDataTypeStr=boolean
  Logical Operator3 : Logic  Operator=XOR  AllPortsSameDT=off  OutDataTypeStr=boolean
  Done : Outport
  wires:
  CLK/1 -> D Flip-Flop2/2, D Flip-Flop1/2, D Flip-Flop 0/2
  ENBL/1 -> D Flip-Flop1/3, D Flip-Flop2/3, D Flip-Flop 0/3
  Logical Operator3/1 -> D Flip-Flop2/1
  D Flip-Flop2/1 -> Done/1, Logical Operator3/2
  Logical Operator1/1 -> Logical Operator3/1
  Logical Operator/1 -> D Flip-Flop1/1
  D Flip-Flop1/1 -> Logical Operator/2, Logical Operator1/2
  D Flip-Flop 0/1 -> Logical Operator/1, Logical Operator1/1
  D Flip-Flop 0/2 -> D Flip-Flop 0/1

== system Logic_Final_Project_PRODUCT4_QUESTION37/Implemention 3/Machine_M4 ==
  ENBL : Inport
  CLK : Inport  Port=2
  D Flip-Flop 0 : simulink_extras/Flip Flops/D Flip-Flop
  D Flip-Flop1 : simulink_extras/Flip Flops/D Flip-Flop
  D Flip-Flop2 : simulink_extras/Flip Flops/D Flip-Flop
  Logical Operator : Logic  Operator=XOR  AllPortsSameDT=off  OutDataTypeStr=boolean
  Logical Operator1 : Logic  AllPortsSameDT=off  OutDataTypeStr=boolean
  Logical Operator2 : Logic  AllPortsSameDT=off  OutDataTypeStr=boolean
  Logical Operator3 : Logic  Operator=XOR  AllPortsSameDT=off  OutDataTypeStr=boolean
  Done : Outport
  wires:
  Logical Operator2/1 -> Done/1
  CLK/1 -> D Flip-Flop2/2, D Flip-Flop1/2, D Flip-Flop 0/2
  ENBL/1 -> D Flip-Flop1/3, D Flip-Flop2/3, D Flip-Flop 0/3
  Logical Operator3/1 -> D Flip-Flop2/1
  D Flip-Flop2/1 -> Logical Operator3/2, Logical Operator2/2
  Logical Operator1/1 -> Logical Operator3/1
  Logical Operator/1 -> D Flip-Flop1/1
  D Flip-Flop1/1 -> Logical Operator/2, Logical Operator1/2
  D Flip-Flop 0/1 -> Logical Operator2/1, Logical Operator/1, Logical Operator1/1
  D Flip-Flop 0/2 -> D Flip-Flop 0/1

== system Logic_Final_Project_PRODUCT4_QUESTION37/Implemention 3/Machine_M6 ==
  ENBL : Inport
  CLK : Inport  Port=2
  D Flip-Flop 0 : simulink_extras/Flip Flops/D Flip-Flop
  D Flip-Flop1 : simulink_extras/Flip Flops/D Flip-Flop
  D Flip-Flop2 : simulink_extras/Flip Flops/D Flip-Flop
  Logical Operator : Logic  Operator=XOR  AllPortsSameDT=off  OutDataTypeStr=boolean
  Logical Operator1 : Logic  AllPortsSameDT=off  OutDataTypeStr=boolean
  Logical Operator2 : Logic  AllPortsSameDT=off  OutDataTypeStr=boolean
  Logical Operator3 : Logic  Operator=XOR  AllPortsSameDT=off  OutDataTypeStr=boolean
  Done : Outport
  wires:
  Logical Operator2/1 -> Done/1
  CLK/1 -> D Flip-Flop2/2, D Flip-Flop1/2, D Flip-Flop 0/2
  ENBL/1 -> D Flip-Flop1/3, D Flip-Flop2/3, D Flip-Flop 0/3
  Logical Operator3/1 -> D Flip-Flop2/1
  D Flip-Flop2/1 -> Logical Operator3/2, Logical Operator2/2
  Logical Operator1/1 -> Logical Operator3/1
  Logical Operator/1 -> D Flip-Flop1/1
  D Flip-Flop1/1 -> Logical Operator/2, Logical Operator1/2, Logical Operator2/1
  D Flip-Flop 0/1 -> Logical Operator/1, Logical Operator1/1
  D Flip-Flop 0/2 -> D Flip-Flop 0/1

== system Logic_Final_Project_PRODUCT4_QUESTION37/Implemention 3/Machine_M7 ==
  ENBL : Inport
  CLK : Inport  Port=2
  D Flip-Flop 0 : simulink_extras/Flip Flops/D Flip-Flop
  D Flip-Flop1 : simulink_extras/Flip Flops/D Flip-Flop
  D Flip-Flop2 : simulink_extras/Flip Flops/D Flip-Flop
  Logical Operator : Logic  Operator=XOR  AllPortsSameDT=off  OutDataTypeStr=boolean
  Logical Operator1 : Logic  AllPortsSameDT=off  OutDataTypeStr=boolean
  Logical Operator3 : Logic  Operator=XOR  AllPortsSameDT=off  OutDataTypeStr=boolean
  Done : Outport
  wires:
  D Flip-Flop 0/2 -> D Flip-Flop 0/1
  D Flip-Flop 0/1 -> Logical Operator1/1, Logical Operator/1
  D Flip-Flop1/1 -> Done/1, Logical Operator1/2, Logical Operator/2
  Logical Operator/1 -> D Flip-Flop1/1
  Logical Operator1/1 -> Logical Operator3/1
  D Flip-Flop2/1 -> Logical Operator3/2
  Logical Operator3/1 -> D Flip-Flop2/1
  ENBL/1 -> D Flip-Flop 0/3, D Flip-Flop2/3, D Flip-Flop1/3
  CLK/1 -> D Flip-Flop 0/2, D Flip-Flop1/2, D Flip-Flop2/2

== system Logic_Final_Project_PRODUCT4_QUESTION37/Implemention 2/PLC/D0 ==
  Enable : Inport
  Q0! : Inport  Port=2
  Q0 : Inport  Port=3
  Logical Operator : Logic  AllPortsSameDT=off  OutDataTypeStr=boolean
  Logical Operator1 : Logic  Operator=NOT  AllPortsSameDT=off  OutDataTypeStr=boolean
  Logical Operator2 : Logic  Operator=OR  AllPortsSameDT=off  OutDataTypeStr=boolean
  Logical Operator3 : Logic  AllPortsSameDT=off  OutDataTypeStr=boolean
  D0 : Outport
  wires:
  Logical Operator1/1 -> Logical Operator/2
  Logical Operator/1 -> Logical Operator2/2
  Logical Operator2/1 -> D0/1
  Logical Operator3/1 -> Logical Operator2/1
  Enable/1 -> Logical Operator1/1, Logical Operator3/1
  Q0!/1 -> Logical Operator3/2
  Q0/1 -> Logical Operator/1

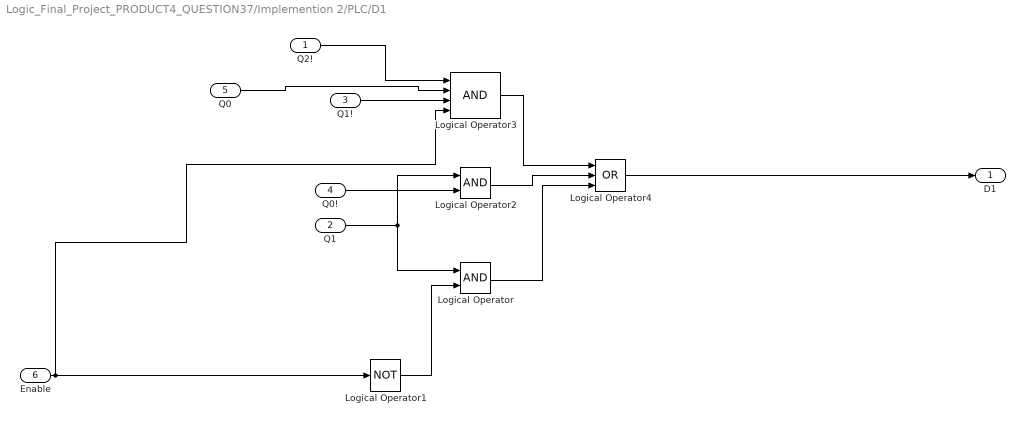
== system Logic_Final_Project_PRODUCT4_QUESTION37/Implemention 2/PLC/D1 ==
  Q2! : Inport
  Q1 : Inport  Port=2
  Q1! : Inport  Port=3
  Q0! : Inport  Port=4
  Q0 : Inport  Port=5
  Enable : Inport  Port=6
  Logical Operator : Logic  AllPortsSameDT=off  OutDataTypeStr=boolean
  Logical Operator1 : Logic  Operator=NOT  AllPortsSameDT=off  OutDataTypeStr=boolean
  Logical Operator2 : Logic  AllPortsSameDT=off  OutDataTypeStr=boolean
  Logical Operator3 : Logic  Inputs=4  AllPortsSameDT=off  OutDataTypeStr=boolean
  Logical Operator4 : Logic  Operator=OR  Inputs=3  AllPortsSameDT=off  OutDataTypeStr=boolean
  D1 : Outport
  wires:
  Q0/1 -> Logical Operator3/2
  Logical Operator1/1 -> Logical Operator/2
  Q1!/1 -> Logical Operator3/3
  Q1/1 -> Logical Operator2/1, Logical Operator/1
  Enable/1 -> Logical Operator3/4, Logical Operator1/1
  Q2!/1 -> Logical Operator3/1
  Q0!/1 -> Logical Operator2/2
  Logical Operator3/1 -> Logical Operator4/1
  Logical Operator2/1 -> Logical Operator4/2
  Logical Operator/1 -> Logical Operator4/3
  Logical Operator4/1 -> D1/1

== system Logic_Final_Project_PRODUCT4_QUESTION37/Implemention 2/PLC/D2  ==
  Q2 : Inport
  Q1 : Inport  Port=2
  Enable : Inport  Port=3
  Q0 : Inport  Port=4
  Q0! : Inport  Port=5
  Logical Operator : Logic  Operator=NOT  AllPortsSameDT=off  OutDataTypeStr=boolean
  Logical Operator1 : Logic  AllPortsSameDT=off  OutDataTypeStr=boolean
  Logical Operator2 : Logic  AllPortsSameDT=off  OutDataTypeStr=boolean
  Logical Operator3 : Logic  Inputs=3  AllPortsSameDT=off  OutDataTypeStr=boolean
  Logical Operator4 : Logic  Operator=OR  Inputs=3  AllPortsSameDT=off  OutDataTypeStr=boolean
  D2 : Outport
  wires:
  Q0/1 -> Logical Operator3/2
  Q2/1 -> Logical Operator2/1, Logical Operator1/1
  Q1/1 -> Logical Operator3/1
  Logical Operator3/1 -> Logical Operator4/3
  Logical Operator/1 -> Logical Operator1/2
  Logical Operator1/1 -> Logical Operator4/2
  Logical Operator2/1 -> Logical Operator4/1
  Enable/1 -> Logical Operator/1, Logical Operator3/3
  Q0!/1 -> Logical Operator2/2
  Logical Operator4/1 -> D2/1

== system Logic_Final_Project_PRODUCT4_QUESTION37/Implemention 3/Machine-M1/Counter_M1 ==
  ENBL : Inport
  CLK : Inport  Port=2
  D Flip-Flop 0 : simulink_extras/Flip Flops/D Flip-Flop
  D Flip-Flop1 : simulink_extras/Flip Flops/D Flip-Flop
  D Flip-Flop2 : simulink_extras/Flip Flops/D Flip-Flop
  Logical Operator : Logic  Operator=XOR  AllPortsSameDT=off  OutDataTypeStr=boolean
  Logical Operator1 : Logic  AllPortsSameDT=off  OutDataTypeStr=boolean
  Logical Operator2 : Logic  AllPortsSameDT=off  OutDataTypeStr=boolean
  Logical Operator3 : Logic  Operator=XOR  AllPortsSameDT=off  OutDataTypeStr=boolean
  Done : Outport
  wires:
  D Flip-Flop 0/2 -> D Flip-Flop 0/1
  D Flip-Flop 0/1 -> Logical Operator1/1, Logical Operator/1, Logical Operator2/1
  D Flip-Flop1/1 -> Logical Operator1/2, Logical Operator/2
  Logical Operator/1 -> D Flip-Flop1/1
  Logical Operator1/1 -> Logical Operator3/1
  D Flip-Flop2/1 -> Logical Operator2/2, Logical Operator3/2
  Logical Operator3/1 -> D Flip-Flop2/1
  ENBL/1 -> D Flip-Flop 0/3, D Flip-Flop2/3, D Flip-Flop1/3
  CLK/1 -> D Flip-Flop 0/2, D Flip-Flop1/2, D Flip-Flop2/2
  Logical Operator2/1 -> Done/1

== system Logic_Final_Project_PRODUCT4_QUESTION37/Implemention 3/Machine-M1/D0 ==
  Enable : Inport
  Q0! : Inport  Port=2
  Q0 : Inport  Port=3
  Logical Operator : Logic  AllPortsSameDT=off  OutDataTypeStr=boolean
  Logical Operator1 : Logic  Operator=NOT  AllPortsSameDT=off  OutDataTypeStr=boolean
  Logical Operator2 : Logic  Operator=OR  AllPortsSameDT=off  OutDataTypeStr=boolean
  Logical Operator3 : Logic  AllPortsSameDT=off  OutDataTypeStr=boolean
  D0 : Outport
  wires:
  Logical Operator1/1 -> Logical Operator/2
  Logical Operator/1 -> Logical Operator2/2
  Logical Operator2/1 -> D0/1
  Logical Operator3/1 -> Logical Operator2/1
  Enable/1 -> Logical Operator1/1, Logical Operator3/1
  Q0!/1 -> Logical Operator3/2
  Q0/1 -> Logical Operator/1

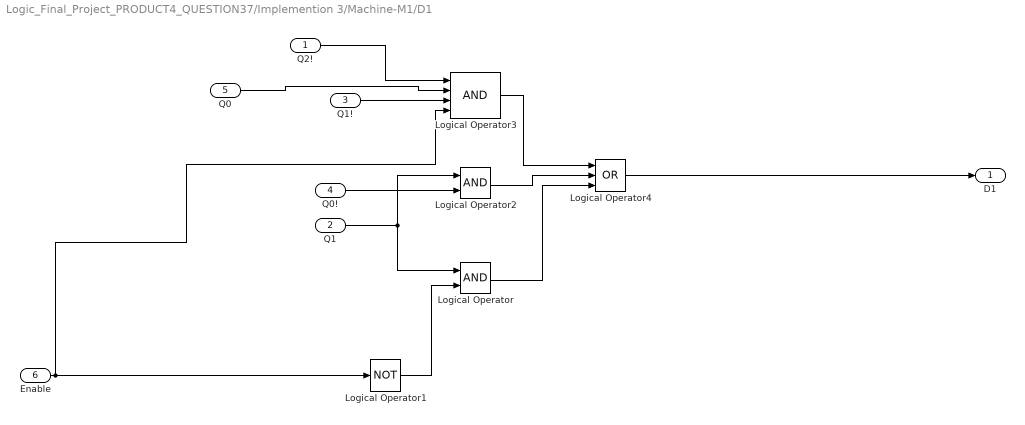
== system Logic_Final_Project_PRODUCT4_QUESTION37/Implemention 3/Machine-M1/D1 ==
  Q2! : Inport
  Q1 : Inport  Port=2
  Q1! : Inport  Port=3
  Q0! : Inport  Port=4
  Q0 : Inport  Port=5
  Enable : Inport  Port=6
  Logical Operator : Logic  AllPortsSameDT=off  OutDataTypeStr=boolean
  Logical Operator1 : Logic  Operator=NOT  AllPortsSameDT=off  OutDataTypeStr=boolean
  Logical Operator2 : Logic  AllPortsSameDT=off  OutDataTypeStr=boolean
  Logical Operator3 : Logic  Inputs=4  AllPortsSameDT=off  OutDataTypeStr=boolean
  Logical Operator4 : Logic  Operator=OR  Inputs=3  AllPortsSameDT=off  OutDataTypeStr=boolean
  D1 : Outport
  wires:
  Q0/1 -> Logical Operator3/2
  Logical Operator1/1 -> Logical Operator/2
  Q1!/1 -> Logical Operator3/3
  Q1/1 -> Logical Operator2/1, Logical Operator/1
  Enable/1 -> Logical Operator3/4, Logical Operator1/1
  Q2!/1 -> Logical Operator3/1
  Q0!/1 -> Logical Operator2/2
  Logical Operator3/1 -> Logical Operator4/1
  Logical Operator2/1 -> Logical Operator4/2
  Logical Operator/1 -> Logical Operator4/3
  Logical Operator4/1 -> D1/1

== system Logic_Final_Project_PRODUCT4_QUESTION37/Implemention 3/Machine-M1/D2  ==
  Q2 : Inport
  Q1 : Inport  Port=2
  Enable : Inport  Port=3
  Q0 : Inport  Port=4
  Q0! : Inport  Port=5
  Logical Operator : Logic  Operator=NOT  AllPortsSameDT=off  OutDataTypeStr=boolean
  Logical Operator1 : Logic  AllPortsSameDT=off  OutDataTypeStr=boolean
  Logical Operator2 : Logic  AllPortsSameDT=off  OutDataTypeStr=boolean
  Logical Operator3 : Logic  Inputs=3  AllPortsSameDT=off  OutDataTypeStr=boolean
  Logical Operator4 : Logic  Operator=OR  Inputs=3  AllPortsSameDT=off  OutDataTypeStr=boolean
  D2 : Outport
  wires:
  Q0/1 -> Logical Operator3/2
  Q2/1 -> Logical Operator2/1, Logical Operator1/1
  Q1/1 -> Logical Operator3/1
  Logical Operator3/1 -> Logical Operator4/3
  Logical Operator/1 -> Logical Operator1/2
  Logical Operator1/1 -> Logical Operator4/2
  Logical Operator2/1 -> Logical Operator4/1
  Enable/1 -> Logical Operator/1, Logical Operator3/3
  Q0!/1 -> Logical Operator2/2
  Logical Operator4/1 -> D2/1

== system Logic_Final_Project_PRODUCT4_QUESTION37/Implemention 3/Machine-M3/D0 ==
  Enable : Inport
  Q0! : Inport  Port=2
  Q0 : Inport  Port=3
  Logical Operator : Logic  AllPortsSameDT=off  OutDataTypeStr=boolean
  Logical Operator1 : Logic  Operator=NOT  AllPortsSameDT=off  OutDataTypeStr=boolean
  Logical Operator2 : Logic  Operator=OR  AllPortsSameDT=off  OutDataTypeStr=boolean
  Logical Operator3 : Logic  AllPortsSameDT=off  OutDataTypeStr=boolean
  D0 : Outport
  wires:
  Q0/1 -> Logical Operator/1
  Q0!/1 -> Logical Operator3/2
  Enable/1 -> Logical Operator3/1, Logical Operator1/1
  Logical Operator3/1 -> Logical Operator2/1
  Logical Operator2/1 -> D0/1
  Logical Operator/1 -> Logical Operator2/2
  Logical Operator1/1 -> Logical Operator/2

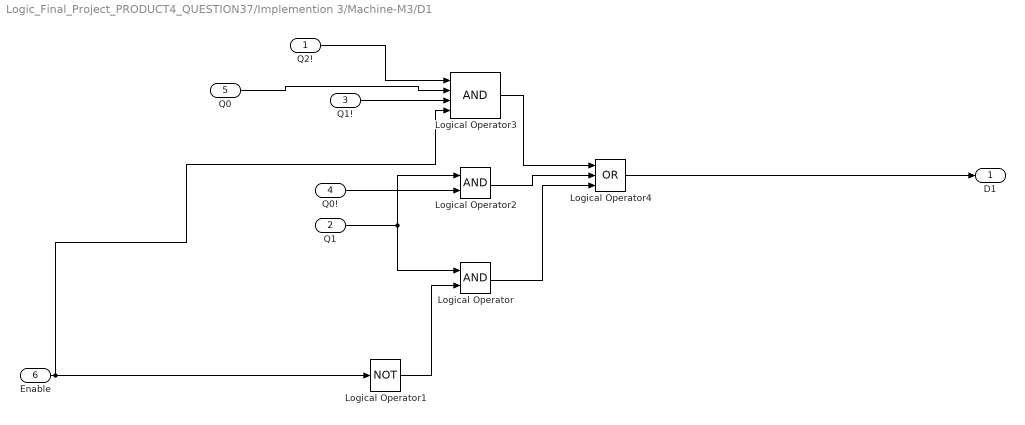
== system Logic_Final_Project_PRODUCT4_QUESTION37/Implemention 3/Machine-M3/D1 ==
  Q2! : Inport
  Q1 : Inport  Port=2
  Q1! : Inport  Port=3
  Q0! : Inport  Port=4
  Q0 : Inport  Port=5
  Enable : Inport  Port=6
  Logical Operator : Logic  AllPortsSameDT=off  OutDataTypeStr=boolean
  Logical Operator1 : Logic  Operator=NOT  AllPortsSameDT=off  OutDataTypeStr=boolean
  Logical Operator2 : Logic  AllPortsSameDT=off  OutDataTypeStr=boolean
  Logical Operator3 : Logic  Inputs=4  AllPortsSameDT=off  OutDataTypeStr=boolean
  Logical Operator4 : Logic  Operator=OR  Inputs=3  AllPortsSameDT=off  OutDataTypeStr=boolean
  D1 : Outport
  wires:
  Logical Operator4/1 -> D1/1
  Logical Operator/1 -> Logical Operator4/3
  Logical Operator2/1 -> Logical Operator4/2
  Logical Operator3/1 -> Logical Operator4/1
  Q0!/1 -> Logical Operator2/2
  Q2!/1 -> Logical Operator3/1
  Enable/1 -> Logical Operator1/1, Logical Operator3/4
  Q1/1 -> Logical Operator/1, Logical Operator2/1
  Q1!/1 -> Logical Operator3/3
  Logical Operator1/1 -> Logical Operator/2
  Q0/1 -> Logical Operator3/2

== system Logic_Final_Project_PRODUCT4_QUESTION37/Implemention 3/Machine-M3/D2  ==
  Q2 : Inport
  Q1 : Inport  Port=2
  Enable : Inport  Port=3
  Q0 : Inport  Port=4
  Q0! : Inport  Port=5
  Logical Operator : Logic  Operator=NOT  AllPortsSameDT=off  OutDataTypeStr=boolean
  Logical Operator1 : Logic  AllPortsSameDT=off  OutDataTypeStr=boolean
  Logical Operator2 : Logic  AllPortsSameDT=off  OutDataTypeStr=boolean
  Logical Operator3 : Logic  Inputs=3  AllPortsSameDT=off  OutDataTypeStr=boolean
  Logical Operator4 : Logic  Operator=OR  Inputs=3  AllPortsSameDT=off  OutDataTypeStr=boolean
  D2 : Outport
  wires:
  Logical Operator4/1 -> D2/1
  Q0!/1 -> Logical Operator2/2
  Enable/1 -> Logical Operator3/3, Logical Operator/1
  Logical Operator2/1 -> Logical Operator4/1
  Logical Operator1/1 -> Logical Operator4/2
  Logical Operator/1 -> Logical Operator1/2
  Logical Operator3/1 -> Logical Operator4/3
  Q1/1 -> Logical Operator3/1
  Q2/1 -> Logical Operator1/1, Logical Operator2/1
  Q0/1 -> Logical Operator3/2

== system Logic_Final_Project_PRODUCT4_QUESTION37/Implemention 3/Machine-M3/Machine_M3 ==
  ENBL : Inport
  CLK : Inport  Port=2
  D Flip-Flop 0 : simulink_extras/Flip Flops/D Flip-Flop
  D Flip-Flop1 : simulink_extras/Flip Flops/D Flip-Flop
  D Flip-Flop2 : simulink_extras/Flip Flops/D Flip-Flop
  Logical Operator : Logic  Operator=XOR  AllPortsSameDT=off  OutDataTypeStr=boolean
  Logical Operator1 : Logic  AllPortsSameDT=off  OutDataTypeStr=boolean
  Logical Operator3 : Logic  Operator=XOR  AllPortsSameDT=off  OutDataTypeStr=boolean
  Done : Outport
  wires:
  CLK/1 -> D Flip-Flop2/2, D Flip-Flop1/2, D Flip-Flop 0/2
  ENBL/1 -> D Flip-Flop1/3, D Flip-Flop2/3, D Flip-Flop 0/3
  Logical Operator3/1 -> D Flip-Flop2/1
  D Flip-Flop2/1 -> Done/1, Logical Operator3/2
  Logical Operator1/1 -> Logical Operator3/1
  Logical Operator/1 -> D Flip-Flop1/1
  D Flip-Flop1/1 -> Logical Operator/2, Logical Operator1/2
  D Flip-Flop 0/1 -> Logical Operator/1, Logical Operator1/1
  D Flip-Flop 0/2 -> D Flip-Flop 0/1

== system Logic_Final_Project_PRODUCT4_QUESTION37/Implemention 3/Machine-M4/D0 ==
  Enable : Inport
  Q0! : Inport  Port=2
  Q0 : Inport  Port=3
  Logical Operator : Logic  AllPortsSameDT=off  OutDataTypeStr=boolean
  Logical Operator1 : Logic  Operator=NOT  AllPortsSameDT=off  OutDataTypeStr=boolean
  Logical Operator2 : Logic  Operator=OR  AllPortsSameDT=off  OutDataTypeStr=boolean
  Logical Operator3 : Logic  AllPortsSameDT=off  OutDataTypeStr=boolean
  D0 : Outport
  wires:
  Logical Operator1/1 -> Logical Operator/2
  Logical Operator/1 -> Logical Operator2/2
  Logical Operator2/1 -> D0/1
  Logical Operator3/1 -> Logical Operator2/1
  Enable/1 -> Logical Operator1/1, Logical Operator3/1
  Q0!/1 -> Logical Operator3/2
  Q0/1 -> Logical Operator/1

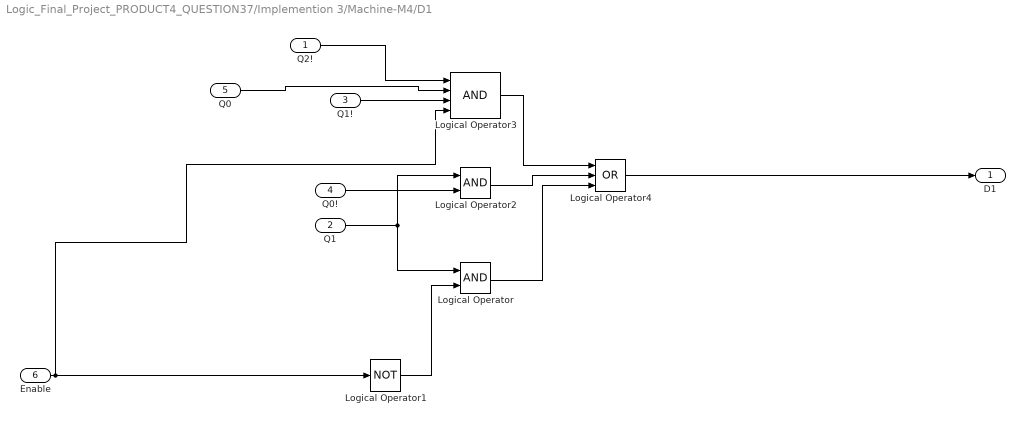
== system Logic_Final_Project_PRODUCT4_QUESTION37/Implemention 3/Machine-M4/D1 ==
  Q2! : Inport
  Q1 : Inport  Port=2
  Q1! : Inport  Port=3
  Q0! : Inport  Port=4
  Q0 : Inport  Port=5
  Enable : Inport  Port=6
  Logical Operator : Logic  AllPortsSameDT=off  OutDataTypeStr=boolean
  Logical Operator1 : Logic  Operator=NOT  AllPortsSameDT=off  OutDataTypeStr=boolean
  Logical Operator2 : Logic  AllPortsSameDT=off  OutDataTypeStr=boolean
  Logical Operator3 : Logic  Inputs=4  AllPortsSameDT=off  OutDataTypeStr=boolean
  Logical Operator4 : Logic  Operator=OR  Inputs=3  AllPortsSameDT=off  OutDataTypeStr=boolean
  D1 : Outport
  wires:
  Q0/1 -> Logical Operator3/2
  Logical Operator1/1 -> Logical Operator/2
  Q1!/1 -> Logical Operator3/3
  Q1/1 -> Logical Operator2/1, Logical Operator/1
  Enable/1 -> Logical Operator3/4, Logical Operator1/1
  Q2!/1 -> Logical Operator3/1
  Q0!/1 -> Logical Operator2/2
  Logical Operator3/1 -> Logical Operator4/1
  Logical Operator2/1 -> Logical Operator4/2
  Logical Operator/1 -> Logical Operator4/3
  Logical Operator4/1 -> D1/1

== system Logic_Final_Project_PRODUCT4_QUESTION37/Implemention 3/Machine-M4/D2  ==
  Q2 : Inport
  Q1 : Inport  Port=2
  Enable : Inport  Port=3
  Q0 : Inport  Port=4
  Q0! : Inport  Port=5
  Logical Operator : Logic  Operator=NOT  AllPortsSameDT=off  OutDataTypeStr=boolean
  Logical Operator1 : Logic  AllPortsSameDT=off  OutDataTypeStr=boolean
  Logical Operator2 : Logic  AllPortsSameDT=off  OutDataTypeStr=boolean
  Logical Operator3 : Logic  Inputs=3  AllPortsSameDT=off  OutDataTypeStr=boolean
  Logical Operator4 : Logic  Operator=OR  Inputs=3  AllPortsSameDT=off  OutDataTypeStr=boolean
  D2 : Outport
  wires:
  Q0/1 -> Logical Operator3/2
  Q2/1 -> Logical Operator2/1, Logical Operator1/1
  Q1/1 -> Logical Operator3/1
  Logical Operator3/1 -> Logical Operator4/3
  Logical Operator/1 -> Logical Operator1/2
  Logical Operator1/1 -> Logical Operator4/2
  Logical Operator2/1 -> Logical Operator4/1
  Enable/1 -> Logical Operator/1, Logical Operator3/3
  Q0!/1 -> Logical Operator2/2
  Logical Operator4/1 -> D2/1

== system Logic_Final_Project_PRODUCT4_QUESTION37/Implemention 3/Machine-M4/Machine_M4 ==
  ENBL : Inport
  CLK : Inport  Port=2
  D Flip-Flop 0 : simulink_extras/Flip Flops/D Flip-Flop
  D Flip-Flop1 : simulink_extras/Flip Flops/D Flip-Flop
  D Flip-Flop2 : simulink_extras/Flip Flops/D Flip-Flop
  Logical Operator : Logic  Operator=XOR  AllPortsSameDT=off  OutDataTypeStr=boolean
  Logical Operator1 : Logic  AllPortsSameDT=off  OutDataTypeStr=boolean
  Logical Operator2 : Logic  AllPortsSameDT=off  OutDataTypeStr=boolean
  Logical Operator3 : Logic  Operator=XOR  AllPortsSameDT=off  OutDataTypeStr=boolean
  Done : Outport
  wires:
  Logical Operator2/1 -> Done/1
  CLK/1 -> D Flip-Flop2/2, D Flip-Flop1/2, D Flip-Flop 0/2
  ENBL/1 -> D Flip-Flop1/3, D Flip-Flop2/3, D Flip-Flop 0/3
  Logical Operator3/1 -> D Flip-Flop2/1
  D Flip-Flop2/1 -> Logical Operator3/2, Logical Operator2/2
  Logical Operator1/1 -> Logical Operator3/1
  Logical Operator/1 -> D Flip-Flop1/1
  D Flip-Flop1/1 -> Logical Operator/2, Logical Operator1/2
  D Flip-Flop 0/1 -> Logical Operator2/1, Logical Operator/1, Logical Operator1/1
  D Flip-Flop 0/2 -> D Flip-Flop 0/1

== system Logic_Final_Project_PRODUCT4_QUESTION37/Implemention 3/Machine-M6/D0 ==
  Enable : Inport
  Q0! : Inport  Port=2
  Q0 : Inport  Port=3
  Logical Operator : Logic  AllPortsSameDT=off  OutDataTypeStr=boolean
  Logical Operator1 : Logic  Operator=NOT  AllPortsSameDT=off  OutDataTypeStr=boolean
  Logical Operator2 : Logic  Operator=OR  AllPortsSameDT=off  OutDataTypeStr=boolean
  Logical Operator3 : Logic  AllPortsSameDT=off  OutDataTypeStr=boolean
  D0 : Outport
  wires:
  Q0/1 -> Logical Operator/1
  Q0!/1 -> Logical Operator3/2
  Enable/1 -> Logical Operator3/1, Logical Operator1/1
  Logical Operator3/1 -> Logical Operator2/1
  Logical Operator2/1 -> D0/1
  Logical Operator/1 -> Logical Operator2/2
  Logical Operator1/1 -> Logical Operator/2
